simulink model "Integrated_Model"  (R2023b)
settings: Solver=ode23s  StartTime=0.0  StopTime=120  FixedStep=0.01  RelTol=1e-3
undefined symbols (not defined in the file): A_sm, A_stack, A_VGS_center, cmp, cp_coolant, ctrl, estNcr, eta_hex, eta_M, J_rotor, k_e_M, k_t_M, lambda, M_H2O, M_Nmix, M_O2, m_st_Nmix_init, m_st_O2_init, m_st_vp_init, p_amb, p_init, R_init, R_M, R_Nmix, R_O2, R_vp, RH_amb, T_amb, T_coolant, T_init, tbn, V_sm, V_stack, V_tbn_m, yO2_amb
libraries: slpidlib x5
(part 1 of 3)
settings Model: Creator=KOTA-Z  LastModifiedBy=KOTA-Z
settings DataIOCC: SaveFinalState=on  SaveOutput=off  DSMLogging=off

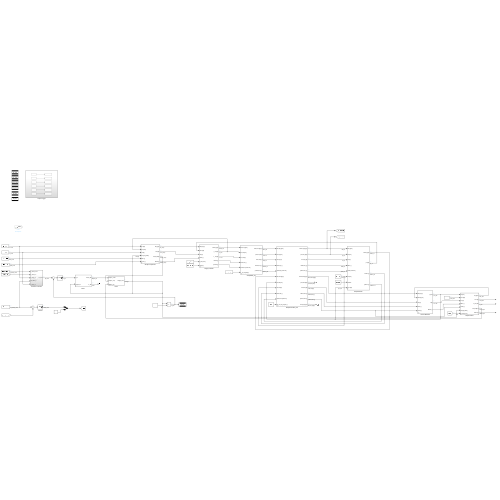
[thumbnail: Simulink's stored preview of the top-level diagram]
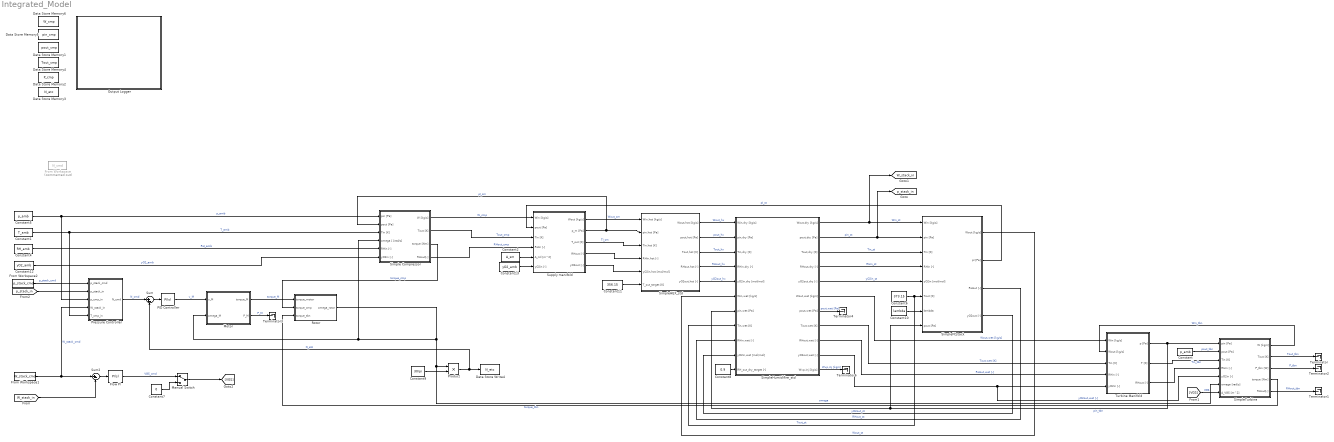
== system Integrated_Model ==
  Constant : Constant  Value=p_amb
  Constant1 : Constant  Value=T_amb
  Constant10 : Constant  Value=lambda
  Constant11 : Constant  Value=356.15
  Constant12 : Constant  Value=yO2_amb
  Constant13 : Constant  Value=yO2_amb
  Constant2 : Constant  Value=A_sm
  Constant4 : Constant  Value=RH_amb
  Constant5 : Constant  Value=p_amb
  Constant6 : Constant  Value=373.15
  Constant7 : Constant  Value=0
  Constant8 : Constant  Value=0.9
  Constant9 : Constant  Value=30/pi
  Data Store Memory1 : DataStoreMemory  DataStoreName=pout_cmp  WriteAfterWriteMsg=warning  ShowAdditionalParam=off
  Data Store Memory2 : DataStoreMemory  DataStoreName=P_cmp  WriteAfterWriteMsg=warning  ShowAdditionalParam=off
  Data Store Memory3 : DataStoreMemory  DataStoreName=N_etc  WriteAfterWriteMsg=warning  ShowAdditionalParam=off
  Data Store Memory4 : DataStoreMemory  DataStoreName=Tout_cmp  WriteAfterWriteMsg=warning  ShowAdditionalParam=off
  Data Store Memory5 : DataStoreMemory  DataStoreName=pin_cmp  WriteAfterWriteMsg=warning  ShowAdditionalParam=off
  Data Store Memory6 : DataStoreMemory  DataStoreName=W_cmp  WriteAfterWriteMsg=warning  ShowAdditionalParam=off
  Data Store Write4 : DataStoreWrite  DataStoreName=N_etc  IndexOptions=Index vector (dialog)  Indices=1  OutputSizes=1
  Flow PI : slpidlib/PID Controller  Controller=PI  Form=Parallel  TimeDomain=Continuous-time  UseExternalTs=off  SampleTime=-1  IntegratorMethod=Forward Euler  FilterMethod=Forward Euler  ControllerParametersSource=internal  P=ctrl.flow.P  I=ctrl.flow.I  UseKiTs=off  D=0  N=100  UseFilter=on  TunerSelectOption=Transfer Function Based (PID Tuner App)  InitialConditionSource=internal  InitialConditionForIntegrator=0  InitialConditionForFilter=0  DifferentiatorICPrevScaledInput=0  ExternalReset=none  TrackingMode=off  Kt=1  LimitOutput=on  SatLimitsSource=internal  UpperSaturationLimit=inf  LowerSaturationLimit=-A_VGS_center  LinearizeAsGain=on  AntiWindupMode=none  Kb=1  LimitIntegrator=off  UpperIntegratorSaturationLimit=inf  LowerIntegratorSaturationLimit=-inf  POutMin=[]  POutMax=[]  IOutMin=[]  IOutMax=[]  DOutMin=[]  DOutMax=[]  NOutMin=[]  NOutMax=[]  SumOutMin=[]  SumOutMax=[]  SaturationOutMin=[]  SaturationOutMax=[]  PParamMin=[]  PParamMax=[]  IParamMin=[]  IParamMax=[]  DParamMin=[]  DParamMax=[]  NParamMin=[]  NParamMax=[]  KbParamMin=[]  KbParamMax=[]  KtParamMin=[]  KtParamMax=[]  KbOutMin=[]  KbOutMax=[]  KtOutMin=[]  KtOutMax=[]  IntegratorOutMin=[]  IntegratorOutMax=[]  FilterOutMin=[]  FilterOutMax=[]  SumI1OutMin=[]  SumI1OutMax=[]  SumI2OutMin=[]  SumI2OutMax=[]  SumI3OutMin=[]  SumI3OutMax=[]  SumI4OutMin=[]  SumI4OutMax=[]  SumDOutMin=[]  SumDOutMax=[]  DifferentiatorOutMin=[]  DifferentiatorOutMax=[]  FilterDiffOutCoefMin=[]  FilterDiffOutCoefMax=[]  ReciprocalOutMin=[]  ReciprocalOutMax=[]  SumDenOutMin=[]  SumDenOutMax=[]  SumNumOutMin=[]  SumNumOutMax=[]  DivideOutMin=[]  DivideOutMax=[]  UdiffTsProdOutMin=[]  UdiffTsProdOutMax=[]  NTsProdOutMin=[]  NTsProdOutMax=[]  UintegralTsProdOutMin=[]  UintegralTsProdOutMax=[]  UngainTsProdOutMin=[]  UngainTsProdOutMax=[]  ClampingZeroOutDataTypeStr=Inherit: Inherit via back propagation  ClampingZeroOutMin=[]  ClampingZeroOutMax=[]  FilterDenConstantOutDataTypeStr=Inherit: Inherit via back propagation  FilterDenConstantOutMin=[]  FilterDenConstantOutMax=[]  PCopyOutDataTypeStr=Inherit: Inherit via back propagation  PCopyOutMin=[]  PCopyOutMax=[]  NCopyOutDataTypeStr=Inherit: Inherit via back propagation  NCopyOutMin=[]  NCopyOutMax=[]  IntegratorContinuousStateAttributes=''  IntegratorStateMustResolveToSignalObject=off  IntegratorRTWStateStorageClass=Auto  FilterContinuousStateAttributes=''  FilterStateMustResolveToSignalObject=off  FilterRTWStateStorageClass=Auto  ParallelPVariant=InternalParameters  IdealPVariant=Disabled  IVariant=InternalParameters  DVariant=Disabled  IntegratorVariant=Continuous  SatVariant=Enabled  AWVariant=Passthrough  PCopyVariant=Disabled  TRVariant=Disabled  FdbkBlocksVariant=Forward  IdealPFdbkVariant=Disabled  SatFdbkVariant=Disabled  DerivativeFilterVariant=Disabled  NVariant=Disabled  NCopyVariant=Disabled_SignalSpec  FilterICVariant=Disabled  IntegratorICVariant=InternalICs  ExternalResetVariant=Disabled  TRSumVariant=Passthrough  SumFdbkVariant=Disabled  SumVariant=Sum_PI  TsampFilterVariant=InternalTs  TsampNgainVariant=Passthrough  TsampIntegralVariant=Disabled_SignalSpec  ExternalSaturationOutDataTypeStr=Inherit: Same as second input
  From Workspace : FromWorkspace  Commented=on  VariableName=N_cmd
  From Workspace1 : FromWorkspace  VariableName=W_stack_cmd
  From Workspace2 : FromWorkspace  VariableName=p_stack_cmd
  Manual Switch : ManualSwitch
  Motor : Subsystem  mask{k_t_M=k_t_M, k_e_M=k_e_M, R_M=R_M, eta_M=eta_M}
      mask prompts: k_t_M "トルク定数 [N*m/A]"; k_e_M "逆起電力係数 [V/(rad/s)]"; R_M "巻線抵抗 [Ω]"; eta_M "モータ機械効率"
      mask DialogControl Parameters Prompt: Motor Parameter
  Output Logger : Subsystem
  PID Controller : slpidlib/PID Controller  Controller=PI  Form=Parallel  TimeDomain=Continuous-time  UseExternalTs=off  SampleTime=-1  IntegratorMethod=Forward Euler  FilterMethod=Forward Euler  ControllerParametersSource=internal  P=ctrl.motor.P  I=ctrl.motor.I  UseKiTs=off  D=0  N=100  UseFilter=on  TunerSelectOption=Transfer Function Based (PID Tuner App)  InitialConditionSource=internal  InitialConditionForIntegrator=0  InitialConditionForFilter=0  DifferentiatorICPrevScaledInput=0  ExternalReset=none  TrackingMode=off  Kt=1  LimitOutput=on  SatLimitsSource=internal  UpperSaturationLimit=500  LowerSaturationLimit=0  LinearizeAsGain=on  AntiWindupMode=none  Kb=1  LimitIntegrator=off  UpperIntegratorSaturationLimit=inf  LowerIntegratorSaturationLimit=-inf  POutMin=[]  POutMax=[]  IOutMin=[]  IOutMax=[]  DOutMin=[]  DOutMax=[]  NOutMin=[]  NOutMax=[]  SumOutMin=[]  SumOutMax=[]  SaturationOutMin=[]  SaturationOutMax=[]  PParamMin=[]  PParamMax=[]  IParamMin=[]  IParamMax=[]  DParamMin=[]  DParamMax=[]  NParamMin=[]  NParamMax=[]  KbParamMin=[]  KbParamMax=[]  KtParamMin=[]  KtParamMax=[]  KbOutMin=[]  KbOutMax=[]  KtOutMin=[]  KtOutMax=[]  IntegratorOutMin=[]  IntegratorOutMax=[]  FilterOutMin=[]  FilterOutMax=[]  SumI1OutMin=[]  SumI1OutMax=[]  SumI2OutMin=[]  SumI2OutMax=[]  SumI3OutMin=[]  SumI3OutMax=[]  SumI4OutMin=[]  SumI4OutMax=[]  SumDOutMin=[]  SumDOutMax=[]  DifferentiatorOutMin=[]  DifferentiatorOutMax=[]  FilterDiffOutCoefMin=[]  FilterDiffOutCoefMax=[]  ReciprocalOutMin=[]  ReciprocalOutMax=[]  SumDenOutMin=[]  SumDenOutMax=[]  SumNumOutMin=[]  SumNumOutMax=[]  DivideOutMin=[]  DivideOutMax=[]  UdiffTsProdOutMin=[]  UdiffTsProdOutMax=[]  NTsProdOutMin=[]  NTsProdOutMax=[]  UintegralTsProdOutMin=[]  UintegralTsProdOutMax=[]  UngainTsProdOutMin=[]  UngainTsProdOutMax=[]  ClampingZeroOutDataTypeStr=Inherit: Inherit via back propagation  ClampingZeroOutMin=[]  ClampingZeroOutMax=[]  FilterDenConstantOutDataTypeStr=Inherit: Inherit via back propagation  FilterDenConstantOutMin=[]  FilterDenConstantOutMax=[]  PCopyOutDataTypeStr=Inherit: Inherit via back propagation  PCopyOutMin=[]  PCopyOutMax=[]  NCopyOutDataTypeStr=Inherit: Inherit via back propagation  NCopyOutMin=[]  NCopyOutMax=[]  IntegratorContinuousStateAttributes=''  IntegratorStateMustResolveToSignalObject=off  IntegratorRTWStateStorageClass=Auto  FilterContinuousStateAttributes=''  FilterStateMustResolveToSignalObject=off  FilterRTWStateStorageClass=Auto  ParallelPVariant=InternalParameters  IdealPVariant=Disabled  IVariant=InternalParameters  DVariant=Disabled  IntegratorVariant=Continuous  SatVariant=Enabled  AWVariant=Passthrough  PCopyVariant=Disabled  TRVariant=Disabled  FdbkBlocksVariant=Forward  IdealPFdbkVariant=Disabled  SatFdbkVariant=Disabled  DerivativeFilterVariant=Disabled  NVariant=Disabled  NCopyVariant=Disabled_SignalSpec  FilterICVariant=Disabled  IntegratorICVariant=InternalICs  ExternalResetVariant=Disabled  TRSumVariant=Passthrough  SumFdbkVariant=Disabled  SumVariant=Sum_PI  TsampFilterVariant=InternalTs  TsampNgainVariant=Passthrough  TsampIntegralVariant=Disabled_SignalSpec  ExternalSaturationOutDataTypeStr=Inherit: Same as second input
  Pressure Controller : Subsystem
  Product : Product
  Rotor : Subsystem  mask{J_rotor=J_rotor}
      mask prompts: J_rotor "Inertia [kg*m^2]"
      mask DialogControl Parameters Prompt: Rotor Parameter
  Simple Compressor : Subsystem  mask{dc=cmp.param.dc, coeff_a=cmp.map.coeff.a, coeff_b=cmp.map.coeff.b, coeff_c=cmp.map.coeff.c, eta_is_cmp=cmp.param.eta_is, eta_m_cmp=cmp.param.eta_mech}
      mask prompts: dc "Inpeller outer diameter"; coeff_a "Map coeffiecient a"; coeff_b "Map coeffiecient b"; coeff_c "Map coeffiecient c"; eta_is_cmp "Isentropic efficiency"; eta_m_cmp "Mechanical efficiency"
      mask DialogControl CmpParameters Prompt: Compressor Parameters
  SimpleFCstack : Subsystem  mask(Simple FCstack){V_ca=V_stack, A_ca=A_stack, R_Nmix=R_Nmix, R_O2=R_O2, R_H2O=R_vp, M_Nmix=M_Nmix, M_O2=M_O2, M_H2O=M_H2O}
      mask prompts: V_ca "Stack Volume (Cathode side) [m^3]"; A_ca "Stack Flow area (Cathode side) [m^2]"; R_Nmix "Gas Constant Nmix [J/kg/K]"; R_O2 "Gas Constant O2 [J/kg/K]"; R_H2O "Gas Constant H2O [J/kg/K]"; M_Nmix "Molecular Weight Nmix [kg/mol]"; M_O2 "Molecular Weight O2 [kg/mol]"; M_H2O "Molecular Weight H2O [kg/mol]"
      mask help: This block provides a simplified FCstack model. The reacted O2 and generated H2O in the stack are calculated based on lambda. Delay due to volume is considered and the pressure drop is approximated as the orifice law.
      mask DialogControl ParameterGroupVar Prompt: Geometric parameter
      mask DialogControl Container3 Prompt: Physical property
  SimpleHEX_std : Subsystem  mask(Simple Heatexchanger){eta_hex=eta_hex, T_cool=T_coolant, cp_cool=cp_coolant}
      mask prompts: eta_hex "Efficiency of HEX [-]"; T_cool "Temperature of coolant [K]"; cp_cool "cp of coolant [J/kg/K]"
      mask help: This block provides a simplified heatexchanger model. Based on the specified thermal efficiency, the exchanged heat is determined.
      mask DialogControl Container3 Prompt: Heatexchanger Parameter
  SimpleHumidifire_std : Subsystem  mask(Simple Humidifire){V_hm=0.1, A_hm=0.1, M_N2=M_Nmix, M_O2=M_O2, M_H2O=M_H2O}
      mask prompts: V_hm "Volume [m^3] (not used)"; A_hm "Flow area [m^2] ] (not used)"; M_N2 "Molecular Weight N2 [kg/mol]"; M_O2 "Molecular Weight O2 [kg/mol]"; M_H2O "Molecular Weight H2O [kg/mol]"
      mask help: This block provides a simplified humidifire model. Depending on the inputed target RH at outlet in dry side, the amount of vapor exchanged between dry and wet side will be calculated. Delay due to volume and pressure drop is not considered.
      mask DialogControl ParameterGroupVar Prompt: Geometric parameter
      mask DialogControl Container3 Prompt: Physical property
  SimpleTurbine : Subsystem  mask{eta_is_tbn=tbn.param.eta_is, eta_m_tbn=tbn.param.eta_mech}
      mask prompts: eta_is_tbn "Isentropic efficiency"; eta_m_tbn "Mechanical efficiency"
      mask DialogControl TbnParameters Prompt: Turbine Parameters
  Sum : Sum  Inputs=|+-
  Sum2 : Sum  Inputs=|+-
  Supply manifold : Subsystem  mask(Supply Manifold){V_m=V_sm, Cd=0.64}
      mask prompts: V_m "Manifold volume [m^3]"; Cd "Discharge coefficient"
      mask help: This block is composed a manifold and a nozzle model.
      mask DialogControl ParameterGroupVar Prompt: Parameter
  Terminator{,1..4,6} (6 alike) : Terminator
  Turbine Manifold : Subsystem  mask{V_m=V_tbn_m}
      mask prompts: V_m "Volume [m^3]"
      mask DialogControl Parameters Prompt: Manifold Parameter
  tag scope: W_stack_in=global, p_stack_in=global
  wires:
  Constant1/1 -> Pressure Controller/5(T_cmp_in), Simple Compressor/3(Tin [K])  "T_amb"
  Constant5/1 -> Pressure Controller/3(p_cmp_in), Simple Compressor/1(pin [Pa])  "p_amb"
  Simple Compressor/1(W [kg/s]) -> Supply manifold/1(Win [kg/s])  "W_cmp"
  Simple Compressor/2(Tout [K]) -> Supply manifold/3(Tin [K])  "Tout_cmp"
  Constant9/1 -> Product/2
  Product/1 -> Sum/2, Data Store Write4/1  "N_etc"
  Rotor/1(omega_rotor) -> Simple Compressor/4(omega [ [rad/s]), Motor/2(omega_M), SimpleTurbine/6(omega [rad/s]), Product/1  "omega"
  Motor/2(P_M) -> Terminator3/1  "P_M"
  Motor/1(torque_M) -> Rotor/1(torque_motor)  "torque_M"
  Simple Compressor/3(torque [Nm]) -> Rotor/2(torque_cmp)  "torque_cmp"
  PID Controller/1 -> Motor/1(v_M)  "v_M"
  Sum/1 -> PID Controller/1
  Constant4/1 -> Simple Compressor/5(RHin [-])  "RH_amb"
  Supply manifold/2(p_m [Pa]) -> SimpleHEX_std/2(pin,hot [Pa]), Simple Compressor/2(pout [Pa])  "pI_sm"
  Constant2/1 -> Supply manifold/5(A_nzl [m^2])
  Simple Compressor/4(RHout[-]) -> Supply manifold/4(RHin [-])  "RHout_cmp"
  SimpleTurbine/1(W [kg/s]) -> Turbine Manifold/2(Wout [kg/s])  "Win_tbn"
  Turbine Manifold/2(T [K]) -> SimpleTurbine/3(Tin [K])  "Tin_tbn"
  Turbine Manifold/1(p [Pa]) -> SimpleFCstack/8(pout [Pa]), SimpleHumidifire_std/7(pin,wet [Pa]), SimpleTurbine/1(pin [Pa])  "pin_tbn"
  Constant/1 -> SimpleTurbine/2(pout [Pa])  "pout_tbn"
  Turbine Manifold/3(RHout [-]) -> SimpleTurbine/4(RHin [-])
  SimpleTurbine/2(Tout [K]) -> Terminator/1  "Tout_tbn"
  SimpleTurbine/5(RHout[-]) -> Terminator1/1  "RHout_tbn"
  SimpleTurbine/3(P_tbn [W]) -> Terminator2/1  "P_tbn"
  Constant10/1 -> SimpleFCstack/7(lambda)
  Supply manifold/1(Wout [kg/s]) -> SimpleHEX_std/1(Win,hot [kg/s])  "Wout_sm"
  Supply manifold/3(T_out [K]) -> SimpleHEX_std/3(Tin,hot [K])  "TI_sm"
  Supply manifold/4(RHout [-]) -> SimpleHEX_std/4(RHin,hot [-])
  SimpleHEX_std/5(yO2out,hot [-]) -> SimpleHumidifire_std/5(yO2in,dry [mol/mol])  "yO2out_hx"
  SimpleHumidifire_std/1(Wout,dry [kg/s]) -> [W_stack_in], SimpleFCstack/1(Win [kg/s])  "Win_st"
  SimpleHumidifire_std/2(pout,dry [Pa]) -> [p_stack_in], SimpleFCstack/2(pin [Pa])  "pin_st"
  SimpleHumidifire_std/3(Tout,dry [K]) -> SimpleFCstack/3(Tin [K])  "Tin_st"
  SimpleHumidifire_std/4(RHout,dry [-]) -> SimpleFCstack/4(RHin [-])  "RHin_st"
  SimpleHumidifire_std/5(yO2out,dry [-]) -> SimpleFCstack/5(yO2in [mol/mol])  "yO2in_st"
  SimpleFCstack/1(Wout [kg/s]) -> SimpleHumidifire_std/6(Win,wet [kg/s])  "Wout_st"
  SimpleFCstack/2(pI [Pa]) -> Supply manifold/2(pout [Pa])  "pI_st"
  Constant6/1 -> SimpleHumidifire_std/8(Tin,wet [K]), SimpleFCstack/6(Tout [K])  "Tout_st"
  SimpleFCstack/3(RHout [-]) -> SimpleHumidifire_std/9(RHin,wet [-])  "RHout_st"
  SimpleFCstack/4(yO2out [-]) -> SimpleHumidifire_std/10(yO2in,wet [mol/mol])  "yO2out_st"
  Constant8/1 -> SimpleHumidifire_std/11(RH_out_dry_target [-])
  SimpleHumidifire_std/6(Wout,wet [kg/s]) -> Turbine Manifold/1(Win [kg/s])  "Wout,wet [kg/s]"
  SimpleHumidifire_std/8(Tout,wet [K]) -> Turbine Manifold/3(Tin [K])  "Tout,wet [K]"
  SimpleHumidifire_std/9(RHout,wet [-]) -> Turbine Manifold/4(RHin [-])  "RHout,wet [-]"
  SimpleTurbine/4(torque [Nm]) -> Rotor/3(torque_tbn)  "torque_tbn"
  SimpleHumidifire_std/7(pout,wet [Pa]) -> Terminator4/1  "pout,wet [Pa]"
  SimpleHumidifire_std/10(yO2out,wet [-]) -> SimpleTurbine/5(yO2in [-]), Turbine Manifold/5(yO2in [-])  "yO2out,wet [-]"
  SimpleHumidifire_std/11(Wvp,inj [kg/s]) -> Terminator6/1  "Wvp,inj [kg/s]"
  Supply manifold/5(yO2out [-]) -> SimpleHEX_std/5(yO2in,hot [mol/mol])
  SimpleHEX_std/3(Tout,hot [K]) -> SimpleHumidifire_std/3(Tin,dry [K])  "Tout_hx"
  SimpleHEX_std/4(RHout,hot [-]) -> SimpleHumidifire_std/4(RHin,dry [-])  "RHout_hx"
  Constant11/1 -> SimpleHEX_std/6(T_out_target [K])
  [VGS] -> SimpleTurbine/7(A_VGS [m^2])  "VGS"
  Sum2/1 -> Flow PI/1
  [W_stack_in] -> Sum2/2
  From Workspace1/1 -> Pressure Controller/4(W_stack_in), Sum2/1  "W_stack_cmd"
  Constant7/1 -> Manual Switch/2
  Manual Switch/1 -> [VGS]
  Flow PI/1 -> Manual Switch/1  "VGS_cmd"
  SimpleHEX_std/1(Wout,hot [kg/s]) -> SimpleHumidifire_std/1(Win,dry [kg/s])  "Wout_hx"
  SimpleHEX_std/2(pout,hot [Pa]) -> SimpleHumidifire_std/2(pin,dry [Pa])  "pout_hx"
  Constant12/1 -> Simple Compressor/6(yO2in [-])  "yO2_amb"
  Constant13/1 -> Supply manifold/6(yO2in [-])
  From Workspace2/1 -> Pressure Controller/1(p_stack_cmd)  "p_stack_cmd"
  [p_stack_in] -> Pressure Controller/2(p_stack_in)
  Pressure Controller/1(N_cmd) -> Sum/1  "N_cmd"

== system Integrated_Model/Motor ==
  v_M : Inport
  omega_M : Inport  Port=2
  Constant : Constant  Value=eta_M*k_t_M/R_M
  Constant1 : Constant  Value=k_e_M
  Minus : Sum  Inputs=+-
  Product : Product
  Product1 : Product
  Product2 : Product
  torque_M : Outport
  P_M : Outport  Port=2
  wires:
  v_M/1 -> Minus/1
  Constant/1 -> Product/2
  Constant1/1 -> Product1/2
  Product1/1 -> Minus/2
  Minus/1 -> Product/1
  omega_M/1 -> Product2/2, Product1/1
  Product/1 -> torque_M/1, Product2/1
  Product2/1 -> P_M/1

== system Integrated_Model/Output Logger ==
  Data Store Read : DataStoreRead  DataStoreName=pin_cmp  IndexOptions=Index vector (dialog)  Indices=1  OutputSizes=1
  Data Store Read1 : DataStoreRead  DataStoreName=W_cmp  IndexOptions=Index vector (dialog)  Indices=1  OutputSizes=1
  Data Store Read2 : DataStoreRead  DataStoreName=Tout_cmp  IndexOptions=Index vector (dialog)  Indices=1  OutputSizes=1
  Data Store Read3 : DataStoreRead  DataStoreName=N_etc  IndexOptions=Index vector (dialog)  Indices=1  OutputSizes=1
  Data Store Read4 : DataStoreRead  DataStoreName=pout_cmp  IndexOptions=Index vector (dialog)  Indices=1  OutputSizes=1
  Data Store Read5 : DataStoreRead  DataStoreName=P_cmp  IndexOptions=Index vector (dialog)  Indices=1  OutputSizes=1
  To Workspace : ToWorkspace  VariableName=pin_cmp  SaveFormat=Timeseries  SampleTime=-1
  To Workspace1 : ToWorkspace  VariableName=pout_cmp  SaveFormat=Timeseries  SampleTime=-1
  To Workspace2 : ToWorkspace  VariableName=W_cmp  SaveFormat=Timeseries  SampleTime=-1
  To Workspace3 : ToWorkspace  VariableName=N_etc  SaveFormat=Timeseries  SampleTime=-1
  To Workspace4 : ToWorkspace  VariableName=Tout_cmp  SaveFormat=Timeseries  SampleTime=-1
  To Workspace5 : ToWorkspace  VariableName=P_cmp  SaveFormat=Timeseries  SampleTime=-1
  wires:
  Data Store Read/1 -> To Workspace/1  "pin_cmp"
  Data Store Read2/1 -> To Workspace4/1
  Data Store Read1/1 -> To Workspace2/1
  Data Store Read4/1 -> To Workspace1/1
  Data Store Read3/1 -> To Workspace3/1
  Data Store Read5/1 -> To Workspace5/1

== system Integrated_Model/Pressure Controller ==
  p_stack_cmd : Inport
  p_stack_in : Inport  Port=2
  p_cmp_in : Inport  Port=3
  W_stack_in : Inport  Port=4
  T_cmp_in : Inport  Port=5
  Display : Display
  Display1 : Display
  Display2 : Display
  Divide : Product  Inputs=*/
  MATLAB Function : MATLAB Function  TreatAsAtomicUnit=on  mask{Ncr_table=estNcr.Ncr_table, Wcr_table=estNcr.Wcr_table, PR_table=estNcr.PR_table}
      mask prompts: Ncr_table "Ncr table [rpm]"; Wcr_table "Wcr table [kg/s]"; PR_table "PR table"
  MATLAB Function1 : MATLAB Function  TreatAsAtomicUnit=on  mask{pref=cmp.ref.p, Tref=cmp.ref.T}
      mask prompts: pref "Refference pressure [Pa]"; Tref "Refference temperature [Pa]"
  MATLAB Function2 : MATLAB Function  TreatAsAtomicUnit=on  mask{Tref=cmp.ref.T}
      mask prompts: Tref "Refference temperature [Pa]"
  Pressure PI : slpidlib/PID Controller  Controller=PI  Form=Parallel  TimeDomain=Continuous-time  UseExternalTs=off  SampleTime=-1  IntegratorMethod=Forward Euler  FilterMethod=Forward Euler  ControllerParametersSource=internal  P=ctrl.pressure.P  I=ctrl.pressure.I  UseKiTs=off  D=0  N=100  UseFilter=on  TunerSelectOption=Transfer Function Based (PID Tuner App)  InitialConditionSource=internal  InitialConditionForIntegrator=0  InitialConditionForFilter=0  DifferentiatorICPrevScaledInput=0  ExternalReset=none  TrackingMode=off  Kt=1  LimitOutput=on  SatLimitsSource=internal  UpperSaturationLimit=20e3  LowerSaturationLimit=-20e3  LinearizeAsGain=on  AntiWindupMode=back-calculation  Kb=1  LimitIntegrator=off  UpperIntegratorSaturationLimit=inf  LowerIntegratorSaturationLimit=-inf  POutMin=[]  POutMax=[]  IOutMin=[]  IOutMax=[]  DOutMin=[]  DOutMax=[]  NOutMin=[]  NOutMax=[]  SumOutMin=[]  SumOutMax=[]  SaturationOutMin=[]  SaturationOutMax=[]  PParamMin=[]  PParamMax=[]  IParamMin=[]  IParamMax=[]  DParamMin=[]  DParamMax=[]  NParamMin=[]  NParamMax=[]  KbParamMin=[]  KbParamMax=[]  KtParamMin=[]  KtParamMax=[]  KbOutMin=[]  KbOutMax=[]  KtOutMin=[]  KtOutMax=[]  IntegratorOutMin=[]  IntegratorOutMax=[]  FilterOutMin=[]  FilterOutMax=[]  SumI1OutMin=[]  SumI1OutMax=[]  SumI2OutMin=[]  SumI2OutMax=[]  SumI3OutMin=[]  SumI3OutMax=[]  SumI4OutMin=[]  SumI4OutMax=[]  SumDOutMin=[]  SumDOutMax=[]  DifferentiatorOutMin=[]  DifferentiatorOutMax=[]  FilterDiffOutCoefMin=[]  FilterDiffOutCoefMax=[]  ReciprocalOutMin=[]  ReciprocalOutMax=[]  SumDenOutMin=[]  SumDenOutMax=[]  SumNumOutMin=[]  SumNumOutMax=[]  DivideOutMin=[]  DivideOutMax=[]  UdiffTsProdOutMin=[]  UdiffTsProdOutMax=[]  NTsProdOutMin=[]  NTsProdOutMax=[]  UintegralTsProdOutMin=[]  UintegralTsProdOutMax=[]  UngainTsProdOutMin=[]  UngainTsProdOutMax=[]  ClampingZeroOutDataTypeStr=Inherit: Inherit via back propagation  ClampingZeroOutMin=[]  ClampingZeroOutMax=[]  FilterDenConstantOutDataTypeStr=Inherit: Inherit via back propagation  FilterDenConstantOutMin=[]  FilterDenConstantOutMax=[]  PCopyOutDataTypeStr=Inherit: Inherit via back propagation  PCopyOutMin=[]  PCopyOutMax=[]  NCopyOutDataTypeStr=Inherit: Inherit via back propagation  NCopyOutMin=[]  NCopyOutMax=[]  IntegratorContinuousStateAttributes=''  IntegratorStateMustResolveToSignalObject=off  IntegratorRTWStateStorageClass=Auto  FilterContinuousStateAttributes=''  FilterStateMustResolveToSignalObject=off  FilterRTWStateStorageClass=Auto  ParallelPVariant=InternalParameters  IdealPVariant=Disabled  IVariant=InternalParameters  DVariant=Disabled  IntegratorVariant=Continuous  SatVariant=Enabled  AWVariant=BackCalculation  PCopyVariant=Disabled  TRVariant=Disabled  FdbkBlocksVariant=Forward  IdealPFdbkVariant=Disabled  SatFdbkVariant=Disabled  DerivativeFilterVariant=Disabled  NVariant=Disabled  NCopyVariant=Disabled_SignalSpec  FilterICVariant=Disabled  IntegratorICVariant=InternalICs  ExternalResetVariant=Disabled  TRSumVariant=Passthrough  SumFdbkVariant=Disabled  SumVariant=Sum_PI  TsampFilterVariant=InternalTs  TsampNgainVariant=Passthrough  TsampIntegralVariant=Disabled_SignalSpec  ExternalSaturationOutDataTypeStr=Inherit: Same as second input
  Sum : Sum  Inputs=|++
  Sum1 : Sum  Inputs=|+-
  N_cmd : Outport
  wires:
  p_stack_in/1 -> Sum1/2
  Sum1/1 -> Pressure PI/1
  Sum/1 -> N_cmd/1
  p_stack_cmd/1 -> Divide/1, Sum1/1
  MATLAB Function1/1(Wcr) -> MATLAB Function/1(Wcr_target), Display2/1
  Divide/1 -> Display1/1, MATLAB Function/2(PR_target)
  MATLAB Function/1(Ncr_est) -> MATLAB Function2/1(Ncr), Display/1
  p_cmp_in/1 -> Divide/2, MATLAB Function1/3(pin)
  W_stack_in/1 -> MATLAB Function1/1(Wact)
  T_cmp_in/1 -> MATLAB Function2/2(Tin), MATLAB Function1/2(Tin)
  Pressure PI/1 -> Sum/1  "N_cmd_FB"
  MATLAB Function2/1(Nact) -> Sum/2  "N_cmd_FF"

== system Integrated_Model/Rotor ==
  torque_motor : Inport
  torque_cmp : Inport  Port=2
  torque_tbn : Inport  Port=3
  Constant : Constant  Value=J_rotor
  Divide : Product  Inputs=*/
  Integrator : Integrator
  Minus : Sum  Inputs=+-+
  omega_rotor : Outport
  wires:
  Constant/1 -> Divide/2
  Divide/1 -> Integrator/1  "dω/dt"
  Integrator/1 -> omega_rotor/1
  torque_motor/1 -> Minus/1
  Minus/1 -> Divide/1
  torque_cmp/1 -> Minus/2
  torque_tbn/1 -> Minus/3

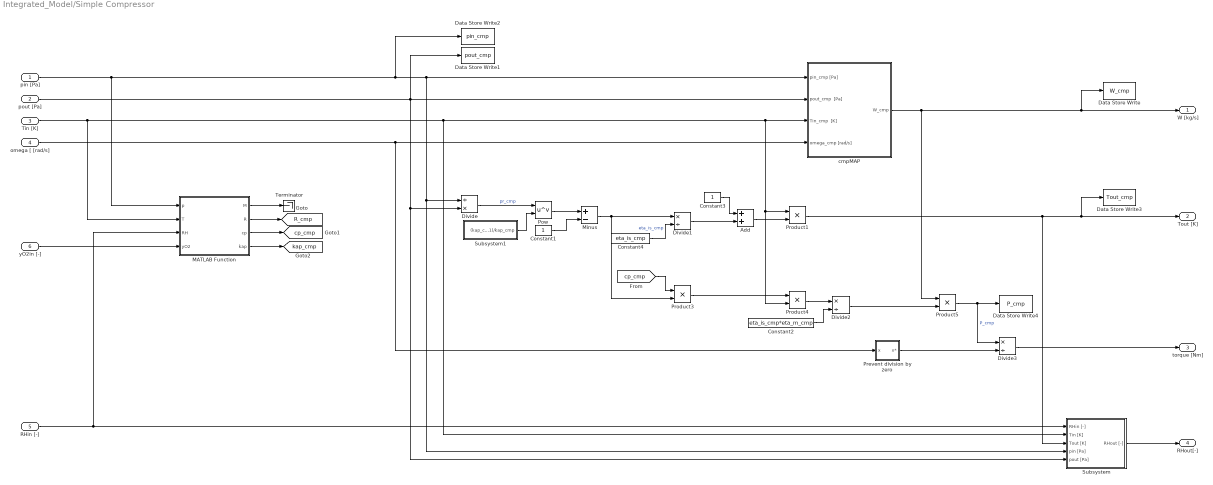
== system Integrated_Model/Simple Compressor ==
  pin [Pa] : Inport
  pout [Pa] : Inport  Port=2
  Tin [K] : Inport  Port=3
  omega [ [rad/s] : Inport  Port=4
  RHin [-] : Inport  Port=5
  yO2in [-] : Inport  Port=6
  Add : Sum
  Constant1 : Constant
  Constant2 : Constant  Value=eta_is_cmp*eta_m_cmp
  Constant3 : Constant
  Constant4 : Constant  Value=eta_is_cmp
  Data Store Write : DataStoreWrite  DataStoreName=W_cmp  IndexOptions=Index vector (dialog)  Indices=1  OutputSizes=1
  Data Store Write1 : DataStoreWrite  DataStoreName=pout_cmp  IndexOptions=Index vector (dialog)  Indices=1  OutputSizes=1
  Data Store Write2 : DataStoreWrite  DataStoreName=pin_cmp  IndexOptions=Index vector (dialog)  Indices=1  OutputSizes=1
  Data Store Write3 : DataStoreWrite  DataStoreName=Tout_cmp  IndexOptions=Index vector (dialog)  Indices=1  OutputSizes=1
  Data Store Write4 : DataStoreWrite  DataStoreName=P_cmp  IndexOptions=Index vector (dialog)  Indices=1  OutputSizes=1
  Divide : Product  Inputs=/*
  Divide1 : Product  Inputs=*/
  Divide2 : Product  Inputs=*/
  Divide3 : Product  Inputs=*/
  MATLAB Function : MATLAB Function  TreatAsAtomicUnit=on  mask{M_O2=M_O2, M_Nmix=M_Nmix, M_H2O=M_H2O}
      mask prompts: M_O2 "Molar mass O2 [kg/mol]"; M_Nmix "Molar mass Nmix [kg/mol]"; M_H2O "Molar mass H2O [kg/mol]"
  Minus : Sum  Inputs=+-
  Pow : Math  Operator=pow  RndMeth=Zero
  Prevent division by zero : Subsystem
  Product{1,3..5} (4 alike) : Product
  Subsystem : Subsystem
  Subsystem1 : Subsystem
  Terminator : Terminator
  cmpMAP : Subsystem
  W [kg/s] : Outport
  Tout [K] : Outport  Port=2
  torque [Nm] : Outport  Port=3
  RHout[-] : Outport  Port=4
  tag scope: R_cmp=global, cp_cmp=global, kap_cmp=global
  wires:
  Divide/1 -> Pow/1  "pr_cmp"
  Subsystem1/1((kap_cmp-1)/kap_cmp) -> Pow/2
  Pow/1 -> Minus/1
  Minus/1 -> Divide1/1, Product3/2
  Constant4/1 -> Divide1/2  "eta_is_cmp"
  Divide1/1 -> Add/2
  Constant3/1 -> Add/1
  Add/1 -> Product1/2
  Tin [K]/1 -> MATLAB Function/2(T), cmpMAP/3(Tin_cmp  [K]), Product4/2, Product1/1, Subsystem/2(Tin [K])
  Constant1/1 -> Minus/2
  [cp_cmp] -> Product3/1
  Product3/1 -> Product4/1
  Product4/1 -> Divide2/1
  Constant2/1 -> Divide2/2
  Divide2/1 -> Product5/2
  Product5/1 -> Data Store Write4/1, Divide3/1  "P_cmp"
  omega [ [rad/s]/1 -> cmpMAP/4(omega_cmp [rad/s]), Prevent division by zero/1(x)
  Prevent division by zero/1(x*) -> Divide3/2
  Divide3/1 -> torque [Nm]/1
  Subsystem/1(RHout [-]) -> RHout[-]/1
  pout [Pa]/1 -> Data Store Write1/1, cmpMAP/2(pout_cmp  [Pa]), Divide/2, Subsystem/5(pout [Pa])
  pin [Pa]/1 -> MATLAB Function/1(p), cmpMAP/1(pin_cmp [Pa]), Divide/1, Subsystem/4(pin [Pa]), Data Store Write2/1
  MATLAB Function/2(R) -> [R_cmp]
  MATLAB Function/3(cp) -> [cp_cmp]
  MATLAB Function/4(kap) -> [kap_cmp]
  MATLAB Function/1(M) -> Terminator/1
  yO2in [-]/1 -> MATLAB Function/4(yO2)
  RHin [-]/1 -> MATLAB Function/3(RH), Subsystem/1(RHin [-])
  cmpMAP/1(W_cmp) -> Product5/1, Data Store Write/1, W [kg/s]/1
  Product1/1 -> Subsystem/3(Tout [K]), Data Store Write3/1, Tout [K]/1

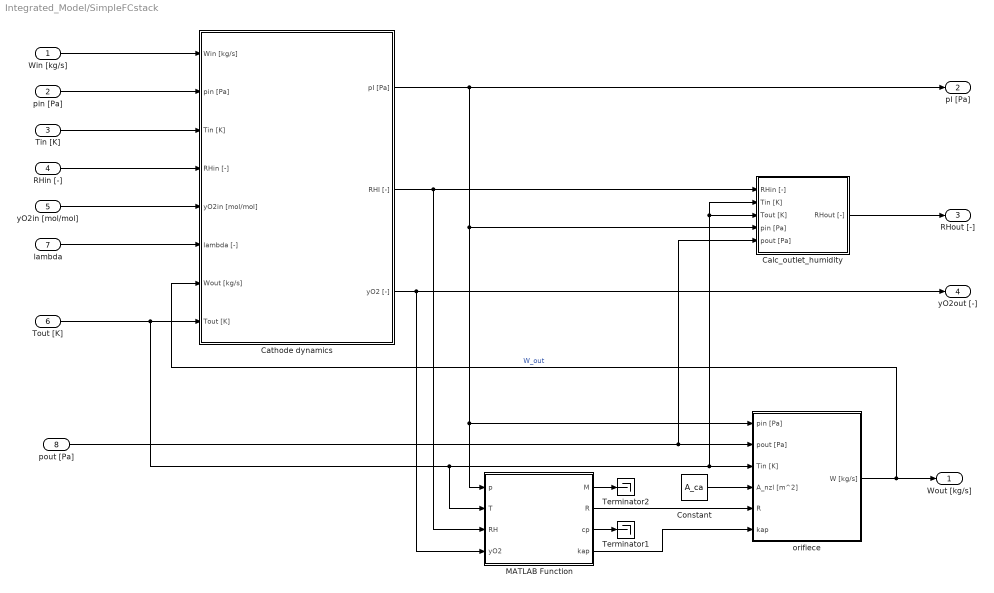
== system Integrated_Model/SimpleFCstack ==
  Win [kg/s] : Inport
  pin [Pa] : Inport  Port=2
  Tin [K] : Inport  Port=3
  RHin [-] : Inport  Port=4
  yO2in [mol/mol] : Inport  Port=5
  Tout [K] : Inport  Port=6
  lambda : Inport  Port=7
  pout [Pa] : Inport  Port=8
  Calc_outlet_humidity : Subsystem
  Cathode dynamics : Subsystem
  Constant : Constant  Value=A_ca
  MATLAB Function : MATLAB Function  TreatAsAtomicUnit=on  mask{M_O2=M_O2, M_Nmix=M_Nmix, M_H2O=M_H2O}
      mask prompts: M_O2 "Molar mass O2 [kg/mol]"; M_Nmix "Molar mass Nmix [kg/mol]"; M_H2O "Molar mass H2O [kg/mol]"
  Terminator1 : Terminator
  Terminator2 : Terminator
  orifiece : Subsystem  mask{Cd_nzl=0.64}
      mask prompts: Cd_nzl "Discharge coefficient"
      mask DialogControl Parameters Prompt: Manifold Parameter
  Wout [kg/s] : Outport
  pI [Pa] : Outport  Port=2
  RHout [-] : Outport  Port=3
  yO2out [-] : Outport  Port=4
  wires:
  pout [Pa]/1 -> orifiece/2(pout [Pa]), Calc_outlet_humidity/5(pout [Pa])
  orifiece/1(W [kg/s]) -> Cathode dynamics/7(Wout [kg/s]), Wout [kg/s]/1  "W_out"
  Constant/1 -> orifiece/4(A_nzl [m^2])
  Cathode dynamics/3(yO2 [-]) -> MATLAB Function/4(yO2), yO2out [-]/1
  Win [kg/s]/1 -> Cathode dynamics/1(Win [kg/s])
  pin [Pa]/1 -> Cathode dynamics/2(pin [Pa])
  lambda/1 -> Cathode dynamics/6(lambda [-])
  Tin [K]/1 -> Cathode dynamics/3(Tin [K])
  RHin [-]/1 -> Cathode dynamics/4(RHin [-])
  Cathode dynamics/1(pI [Pa]) -> pI [Pa]/1, Calc_outlet_humidity/4(pin [Pa]), MATLAB Function/1(p), orifiece/1(pin [Pa])
  yO2in [mol/mol]/1 -> Cathode dynamics/5(yO2in [mol/mol])
  Tout [K]/1 -> MATLAB Function/2(T), Calc_outlet_humidity/3(Tout [K]), Calc_outlet_humidity/2(Tin [K]), orifiece/3(Tin [K]), Cathode dynamics/8(Tout [K])
  Calc_outlet_humidity/1(RHout [-]) -> RHout [-]/1
  MATLAB Function/4(kap) -> orifiece/6(kap)
  MATLAB Function/1(M) -> Terminator2/1
  MATLAB Function/3(cp) -> Terminator1/1
  MATLAB Function/2(R) -> orifiece/5(R)
  Cathode dynamics/2(RHI [-]) -> MATLAB Function/3(RH), Calc_outlet_humidity/1(RHin [-])

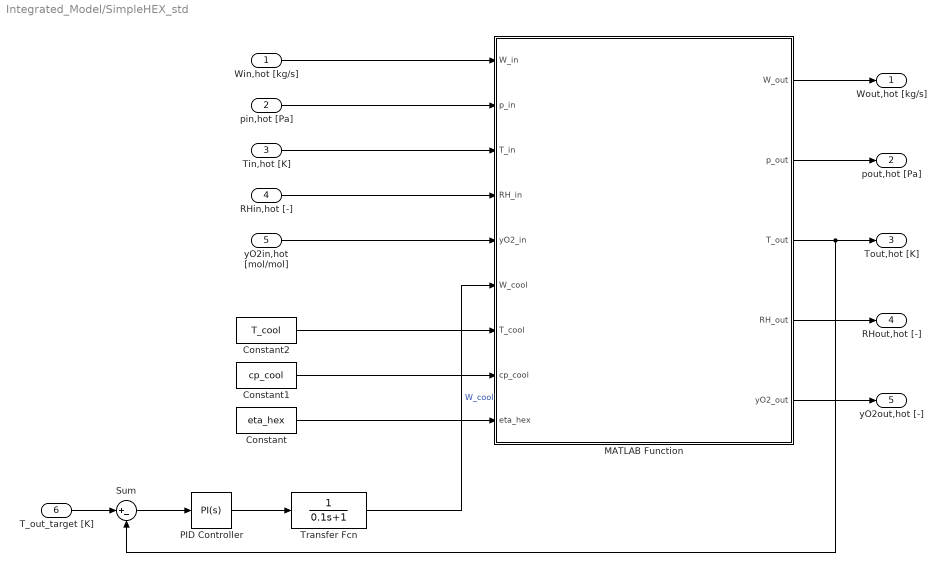
== system Integrated_Model/SimpleHEX_std ==
  Win,hot [kg/s] : Inport
  pin,hot [Pa] : Inport  Port=2
  Tin,hot [K] : Inport  Port=3
  RHin,hot [-] : Inport  Port=4
  yO2in,hot [mol/mol] : Inport  Port=5
  T_out_target [K] : Inport  Port=6
  Constant : Constant  Value=eta_hex
  Constant1 : Constant  Value=cp_cool
  Constant2 : Constant  Value=T_cool
  MATLAB Function : MATLAB Function  TreatAsAtomicUnit=on  mask{M_O2=M_O2, M_Nmix=M_Nmix, M_H2O=M_H2O}
      mask prompts: M_O2 "Molar mass O2 [kg/mol]"; M_Nmix "Molar mass Nmix [kg/mol]"; M_H2O "Molar mass H2O [kg/mol]"
  PID Controller : slpidlib/PID Controller  Controller=PI  Form=Parallel  TimeDomain=Continuous-time  UseExternalTs=off  SampleTime=-1  IntegratorMethod=Forward Euler  FilterMethod=Forward Euler  ControllerParametersSource=internal  P=-0.01  I=-0.1  UseKiTs=off  D=0  N=100  UseFilter=on  TunerSelectOption=Transfer Function Based (PID Tuner App)  InitialConditionSource=internal  InitialConditionForIntegrator=0  InitialConditionForFilter=0  DifferentiatorICPrevScaledInput=0  ExternalReset=none  TrackingMode=off  Kt=1  LimitOutput=on  SatLimitsSource=internal  UpperSaturationLimit=2  LowerSaturationLimit=0  LinearizeAsGain=on  AntiWindupMode=back-calculation  Kb=1  LimitIntegrator=off  UpperIntegratorSaturationLimit=inf  LowerIntegratorSaturationLimit=-inf  POutMin=[]  POutMax=[]  IOutMin=[]  IOutMax=[]  DOutMin=[]  DOutMax=[]  NOutMin=[]  NOutMax=[]  SumOutMin=[]  SumOutMax=[]  SaturationOutMin=[]  SaturationOutMax=[]  PParamMin=[]  PParamMax=[]  IParamMin=[]  IParamMax=[]  DParamMin=[]  DParamMax=[]  NParamMin=[]  NParamMax=[]  KbParamMin=[]  KbParamMax=[]  KtParamMin=[]  KtParamMax=[]  KbOutMin=[]  KbOutMax=[]  KtOutMin=[]  KtOutMax=[]  IntegratorOutMin=[]  IntegratorOutMax=[]  FilterOutMin=[]  FilterOutMax=[]  SumI1OutMin=[]  SumI1OutMax=[]  SumI2OutMin=[]  SumI2OutMax=[]  SumI3OutMin=[]  SumI3OutMax=[]  SumI4OutMin=[]  SumI4OutMax=[]  SumDOutMin=[]  SumDOutMax=[]  DifferentiatorOutMin=[]  DifferentiatorOutMax=[]  FilterDiffOutCoefMin=[]  FilterDiffOutCoefMax=[]  ReciprocalOutMin=[]  ReciprocalOutMax=[]  SumDenOutMin=[]  SumDenOutMax=[]  SumNumOutMin=[]  SumNumOutMax=[]  DivideOutMin=[]  DivideOutMax=[]  UdiffTsProdOutMin=[]  UdiffTsProdOutMax=[]  NTsProdOutMin=[]  NTsProdOutMax=[]  UintegralTsProdOutMin=[]  UintegralTsProdOutMax=[]  UngainTsProdOutMin=[]  UngainTsProdOutMax=[]  ClampingZeroOutDataTypeStr=Inherit: Inherit via back propagation  ClampingZeroOutMin=[]  ClampingZeroOutMax=[]  FilterDenConstantOutDataTypeStr=Inherit: Inherit via back propagation  FilterDenConstantOutMin=[]  FilterDenConstantOutMax=[]  PCopyOutDataTypeStr=Inherit: Inherit via back propagation  PCopyOutMin=[]  PCopyOutMax=[]  NCopyOutDataTypeStr=Inherit: Inherit via back propagation  NCopyOutMin=[]  NCopyOutMax=[]  IntegratorContinuousStateAttributes=''  IntegratorStateMustResolveToSignalObject=off  IntegratorRTWStateStorageClass=Auto  FilterContinuousStateAttributes=''  FilterStateMustResolveToSignalObject=off  FilterRTWStateStorageClass=Auto  ParallelPVariant=InternalParameters  IdealPVariant=Disabled  IVariant=InternalParameters  DVariant=Disabled  IntegratorVariant=Continuous  SatVariant=Enabled  AWVariant=BackCalculation  PCopyVariant=Disabled  TRVariant=Disabled  FdbkBlocksVariant=Forward  IdealPFdbkVariant=Disabled  SatFdbkVariant=Disabled  DerivativeFilterVariant=Disabled  NVariant=Disabled  NCopyVariant=Disabled_SignalSpec  FilterICVariant=Disabled  IntegratorICVariant=InternalICs  ExternalResetVariant=Disabled  TRSumVariant=Passthrough  SumFdbkVariant=Disabled  SumVariant=Sum_PI  TsampFilterVariant=InternalTs  TsampNgainVariant=Passthrough  TsampIntegralVariant=Disabled_SignalSpec  ExternalSaturationOutDataTypeStr=Inherit: Same as second input
  Sum : Sum  Inputs=|+-
  Transfer Fcn : TransferFcn  Denominator=[0.1 1]
  Wout,hot [kg/s] : Outport
  pout,hot [Pa] : Outport  Port=2
  Tout,hot [K] : Outport  Port=3
  RHout,hot [-] : Outport  Port=4
  yO2out,hot [-] : Outport  Port=5
  wires:
  MATLAB Function/5(yO2_out) -> yO2out,hot [-]/1
  MATLAB Function/2(p_out) -> pout,hot [Pa]/1
  MATLAB Function/1(W_out) -> Wout,hot [kg/s]/1
  MATLAB Function/4(RH_out) -> RHout,hot [-]/1
  MATLAB Function/3(T_out) -> Sum/2, Tout,hot [K]/1
  RHin,hot [-]/1 -> MATLAB Function/4(RH_in)
  pin,hot [Pa]/1 -> MATLAB Function/2(p_in)
  Tin,hot [K]/1 -> MATLAB Function/3(T_in)
  Win,hot [kg/s]/1 -> MATLAB Function/1(W_in)
  yO2in,hot [mol/mol]/1 -> MATLAB Function/5(yO2_in)
  PID Controller/1 -> Transfer Fcn/1
  Transfer Fcn/1 -> MATLAB Function/6(W_cool)  "W_cool"
  Sum/1 -> PID Controller/1
  T_out_target [K]/1 -> Sum/1
  Constant2/1 -> MATLAB Function/7(T_cool)
  Constant1/1 -> MATLAB Function/8(cp_cool)
  Constant/1 -> MATLAB Function/9(eta_hex)

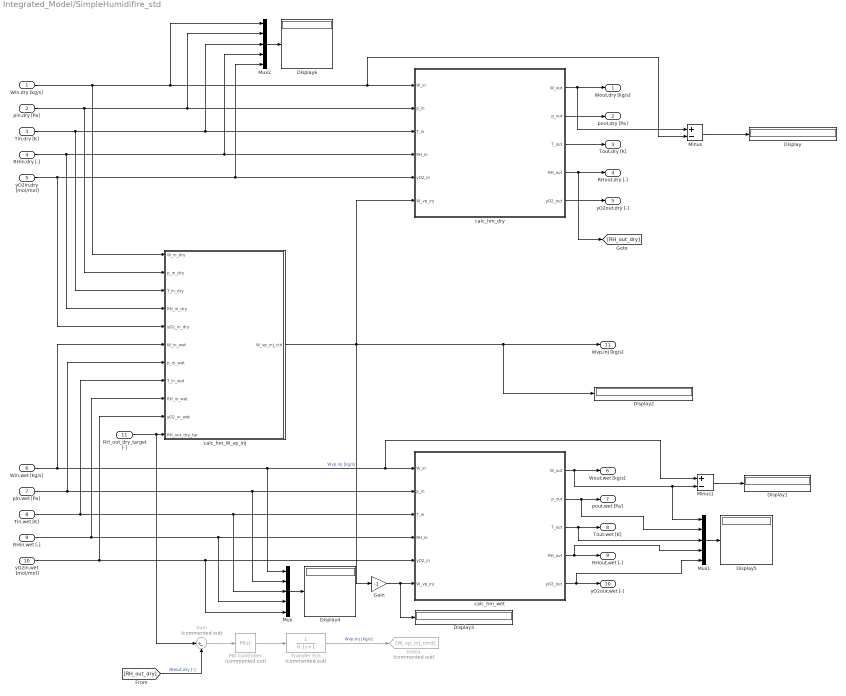
== system Integrated_Model/SimpleHumidifire_std ==
  Win,dry [kg/s] : Inport
  pin,dry [Pa] : Inport  Port=2
  Tin,dry [K] : Inport  Port=3
  RHin,dry [-] : Inport  Port=4
  yO2in,dry [mol/mol] : Inport  Port=5
  Win,wet [kg/s] : Inport  Port=6
  pin,wet [Pa] : Inport  Port=7
  Tin,wet [K] : Inport  Port=8
  RHin,wet [-] : Inport  Port=9
  yO2in,wet [mol/mol] : Inport  Port=10
  RH_out_dry_target [-] : Inport  Port=11
  Display{,1..6} (7 alike) : Display
  Gain : Gain  Gain=-1
  Goto1 : Goto  Commented=on  GotoTag=W_vp_inj_cmd
  Minus : Sum  Inputs=+-
  Minus1 : Sum  Inputs=+-
  Mux : Mux  Inputs=5
  Mux1 : Mux  Inputs=5
  Mux2 : Mux  Inputs=5
  PID Controller : slpidlib/PID Controller  Commented=on  Controller=PI  Form=Parallel  TimeDomain=Continuous-time  UseExternalTs=off  SampleTime=-1  IntegratorMethod=Forward Euler  FilterMethod=Forward Euler  ControllerParametersSource=internal  P=1  I=0.1  UseKiTs=off  D=0  N=100  UseFilter=on  TunerSelectOption=Transfer Function Based (PID Tuner App)  InitialConditionSource=internal  InitialConditionForIntegrator=0  InitialConditionForFilter=0  DifferentiatorICPrevScaledInput=0  ExternalReset=none  TrackingMode=off  Kt=1  LimitOutput=on  SatLimitsSource=internal  UpperSaturationLimit=1  LowerSaturationLimit=0  LinearizeAsGain=on  AntiWindupMode=back-calculation  Kb=1  LimitIntegrator=off  UpperIntegratorSaturationLimit=inf  LowerIntegratorSaturationLimit=-inf  POutMin=[]  POutMax=[]  IOutMin=[]  IOutMax=[]  DOutMin=[]  DOutMax=[]  NOutMin=[]  NOutMax=[]  SumOutMin=[]  SumOutMax=[]  SaturationOutMin=[]  SaturationOutMax=[]  PParamMin=[]  PParamMax=[]  IParamMin=[]  IParamMax=[]  DParamMin=[]  DParamMax=[]  NParamMin=[]  NParamMax=[]  KbParamMin=[]  KbParamMax=[]  KtParamMin=[]  KtParamMax=[]  KbOutMin=[]  KbOutMax=[]  KtOutMin=[]  KtOutMax=[]  IntegratorOutMin=[]  IntegratorOutMax=[]  FilterOutMin=[]  FilterOutMax=[]  SumI1OutMin=[]  SumI1OutMax=[]  SumI2OutMin=[]  SumI2OutMax=[]  SumI3OutMin=[]  SumI3OutMax=[]  SumI4OutMin=[]  SumI4OutMax=[]  SumDOutMin=[]  SumDOutMax=[]  DifferentiatorOutMin=[]  DifferentiatorOutMax=[]  FilterDiffOutCoefMin=[]  FilterDiffOutCoefMax=[]  ReciprocalOutMin=[]  ReciprocalOutMax=[]  SumDenOutMin=[]  SumDenOutMax=[]  SumNumOutMin=[]  SumNumOutMax=[]  DivideOutMin=[]  DivideOutMax=[]  UdiffTsProdOutMin=[]  UdiffTsProdOutMax=[]  NTsProdOutMin=[]  NTsProdOutMax=[]  UintegralTsProdOutMin=[]  UintegralTsProdOutMax=[]  UngainTsProdOutMin=[]  UngainTsProdOutMax=[]  ClampingZeroOutDataTypeStr=Inherit: Inherit via back propagation  ClampingZeroOutMin=[]  ClampingZeroOutMax=[]  FilterDenConstantOutDataTypeStr=Inherit: Inherit via back propagation  FilterDenConstantOutMin=[]  FilterDenConstantOutMax=[]  PCopyOutDataTypeStr=Inherit: Inherit via back propagation  PCopyOutMin=[]  PCopyOutMax=[]  NCopyOutDataTypeStr=Inherit: Inherit via back propagation  NCopyOutMin=[]  NCopyOutMax=[]  IntegratorContinuousStateAttributes=''  IntegratorStateMustResolveToSignalObject=off  IntegratorRTWStateStorageClass=Auto  FilterContinuousStateAttributes=''  FilterStateMustResolveToSignalObject=off  FilterRTWStateStorageClass=Auto  ParallelPVariant=InternalParameters  IdealPVariant=Disabled  IVariant=InternalParameters  DVariant=Disabled  IntegratorVariant=Continuous  SatVariant=Enabled  AWVariant=BackCalculation  PCopyVariant=Disabled  TRVariant=Disabled  FdbkBlocksVariant=Forward  IdealPFdbkVariant=Disabled  SatFdbkVariant=Disabled  DerivativeFilterVariant=Disabled  NVariant=Disabled  NCopyVariant=Disabled_SignalSpec  FilterICVariant=Disabled  IntegratorICVariant=InternalICs  ExternalResetVariant=Disabled  TRSumVariant=Passthrough  SumFdbkVariant=Disabled  SumVariant=Sum_PI  TsampFilterVariant=InternalTs  TsampNgainVariant=Passthrough  TsampIntegralVariant=Disabled_SignalSpec  ExternalSaturationOutDataTypeStr=Inherit: Same as second input
  Sum : Sum  Commented=on  Inputs=|+-
  Transfer Fcn : TransferFcn  Commented=on  Denominator=[0.1 1]
  calc_hm_W_vp_inj : MATLAB Function  TreatAsAtomicUnit=on  mask{M_O2=M_O2, M_Nmix=M_Nmix, M_H2O=M_H2O}
      mask prompts: M_O2 "Molar mass O2 [kg/mol]"; M_Nmix "Molar mass N2 [kg/mol]"; M_H2O "Molar mass H2O [kg/mol]"
  calc_hm_dry : MATLAB Function  TreatAsAtomicUnit=on  mask{M_O2=M_O2, M_Nmix=M_Nmix, M_H2O=M_H2O}
      mask prompts: M_O2 "Molar mass O2 [kg/mol]"; M_Nmix "Molar mass Nmix [kg/mol]"; M_H2O "Molar mass H2O [kg/mol]"
  calc_hm_wet : MATLAB Function  TreatAsAtomicUnit=on  mask{M_O2=M_O2, M_Nmix=M_Nmix, M_H2O=M_H2O}
      mask prompts: M_O2 "Molar mass O2 [kg/mol]"; M_Nmix "Molar mass Nmix [kg/mol]"; M_H2O "Molar mass H2O [kg/mol]"
  Wout,dry [kg/s] : Outport
  pout,dry [Pa] : Outport  Port=2
  Tout,dry [K] : Outport  Port=3
  RHout,dry [-] : Outport  Port=4
  yO2out,dry [-] : Outport  Port=5
  Wout,wet [kg/s] : Outport  Port=6
  pout,wet [Pa] : Outport  Port=7
  Tout,wet [K] : Outport  Port=8
  RHout,wet [-] : Outport  Port=9
  yO2out,wet [-] : Outport  Port=10
  Wvp,inj [kg/s] : Outport  Port=11
  wires:
  calc_hm_dry/5(yO2_out) -> yO2out,dry [-]/1
  calc_hm_dry/2(p_out) -> pout,dry [Pa]/1
  calc_hm_dry/4(RH_out) -> RHout,dry [-]/1, [RH_out_dry]
  calc_hm_dry/3(T_out) -> Tout,dry [K]/1
  pin,wet [Pa]/1 -> Mux/2, calc_hm_wet/2(p_in), calc_hm_W_vp_inj/7(p_in_wet)
  Win,wet [kg/s]/1 -> Mux/1, calc_hm_wet/1(W_in), Minus1/1, calc_hm_W_vp_inj/6(W_in_wet)
  RHin,wet [-]/1 -> Mux/4, calc_hm_wet/4(RH_in), calc_hm_W_vp_inj/9(RH_in_wet)
  yO2in,wet [mol/mol]/1 -> Mux/5, calc_hm_wet/5(yO2_in), calc_hm_W_vp_inj/10(yO2_in_wet)
  Tin,wet [K]/1 -> Mux/3, calc_hm_wet/3(T_in), calc_hm_W_vp_inj/8(T_in_wet)
  calc_hm_wet/1(W_out) -> Mux1/1, Minus1/2, Wout,wet [kg/s]/1
  calc_hm_wet/2(p_out) -> Mux1/2, pout,wet [Pa]/1
  calc_hm_wet/3(T_out) -> Mux1/3, Tout,wet [K]/1
  calc_hm_wet/4(RH_out) -> Mux1/4, RHout,wet [-]/1
  calc_hm_wet/5(yO2_out) -> Mux1/5, yO2out,wet [-]/1
  PID Controller/1 -> Transfer Fcn/1
  Transfer Fcn/1 -> Goto1/1  "Wvp,inj [kg/s]"
  Sum/1 -> PID Controller/1
  RH_out_dry_target [-]/1 -> calc_hm_W_vp_inj/11(RH_out_dry_tar), Sum/1
  [RH_out_dry] -> Sum/2  "RHout,dry [-]"
  Gain/1 -> Display3/1, calc_hm_wet/6(W_vp_inj)
  calc_hm_W_vp_inj/1(W_vp_inj_ctrl) -> calc_hm_dry/6(W_vp_inj), Display2/1, Wvp,inj [kg/s]/1, Gain/1  "Wvp,inj [kg/s]"
  Minus/1 -> Display/1
  calc_hm_dry/1(W_out) -> Minus/1, Wout,dry [kg/s]/1
  Minus1/1 -> Display1/1
  Mux/1 -> Display4/1
  Mux1/1 -> Display5/1
  pin,dry [Pa]/1 -> Mux2/2, calc_hm_dry/2(p_in), calc_hm_W_vp_inj/2(p_in_dry)
  Tin,dry [K]/1 -> Mux2/3, calc_hm_dry/3(T_in), calc_hm_W_vp_inj/3(T_in_dry)
  Win,dry [kg/s]/1 -> Mux2/1, Minus/2, calc_hm_dry/1(W_in), calc_hm_W_vp_inj/1(W_in_dry)
  RHin,dry [-]/1 -> Mux2/4, calc_hm_dry/4(RH_in), calc_hm_W_vp_inj/4(RH_in_dry)
  yO2in,dry [mol/mol]/1 -> Mux2/5, calc_hm_dry/5(yO2_in), calc_hm_W_vp_inj/5(yO2_in_dry)
  Mux2/1 -> Display6/1

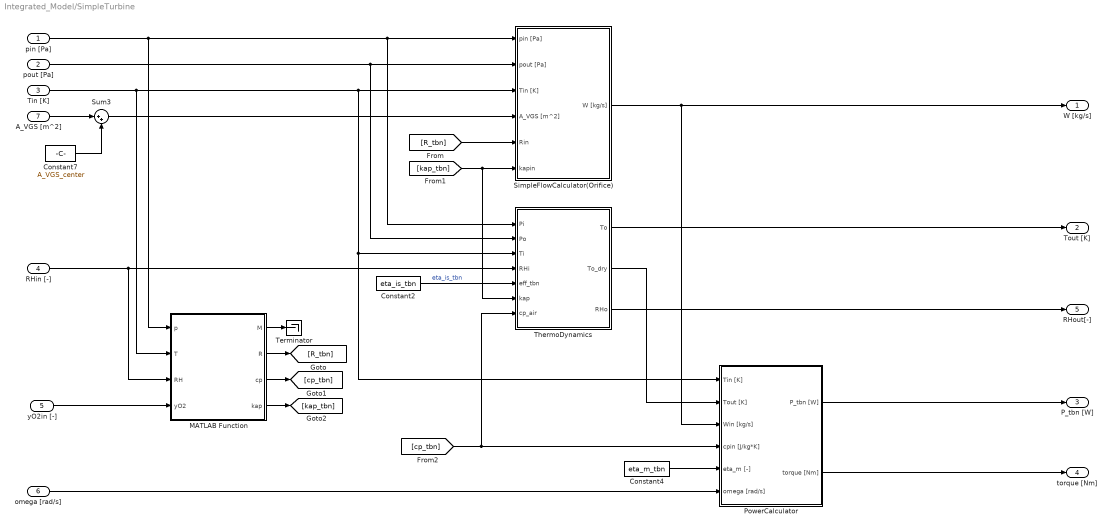
== system Integrated_Model/SimpleTurbine ==
  pin [Pa] : Inport
  pout [Pa] : Inport  Port=2
  Tin [K] : Inport  Port=3
  RHin [-] : Inport  Port=4
  yO2in [-] : Inport  Port=5
  omega [rad/s] : Inport  Port=6
  A_VGS [m^2] : Inport  Port=7
  Constant2 : Constant  Value=eta_is_tbn
  Constant4 : Constant  Value=eta_m_tbn
  Constant7 : Constant  Value=A_VGS_center
  MATLAB Function : MATLAB Function  TreatAsAtomicUnit=on  mask{M_O2=M_O2, M_Nmix=M_Nmix, M_H2O=M_H2O}
      mask prompts: M_O2 "Molar mass O2 [kg/mol]"; M_Nmix "Molar mass Nmix [kg/mol]"; M_H2O "Molar mass H2O [kg/mol]"
  PowerCalculator : Subsystem
  SimpleFlowCalculator(Orifice) : Subsystem
  Sum3 : Sum  Inputs=|++
  Terminator : Terminator
  ThermoDynamics : MATLAB Function  TreatAsAtomicUnit=on
  W [kg/s] : Outport
  Tout [K] : Outport  Port=2
  P_tbn [W] : Outport  Port=3
  torque [Nm] : Outport  Port=4
  RHout[-] : Outport  Port=5
  wires:
  pin [Pa]/1 -> MATLAB Function/1(p), ThermoDynamics/1(Pi), SimpleFlowCalculator(Orifice)/1(pin [Pa])
  Tin [K]/1 -> MATLAB Function/2(T), SimpleFlowCalculator(Orifice)/3(Tin [K]), PowerCalculator/1(Tin [K]), ThermoDynamics/3(Ti)
  SimpleFlowCalculator(Orifice)/1(W [kg/s]) -> PowerCalculator/3(Win [kg/s]), W [kg/s]/1
  pout [Pa]/1 -> ThermoDynamics/2(Po), SimpleFlowCalculator(Orifice)/2(pout [Pa])
  ThermoDynamics/3(RHo) -> RHout[-]/1
  PowerCalculator/1(P_tbn [W]) -> P_tbn [W]/1
  [R_tbn] -> SimpleFlowCalculator(Orifice)/5(Rin)
  [kap_tbn] -> ThermoDynamics/6(kap), SimpleFlowCalculator(Orifice)/6(kapin)
  Constant4/1 -> PowerCalculator/5(eta_m [-])
  omega [rad/s]/1 -> PowerCalculator/6(omega [rad/s])
  PowerCalculator/2(torque [Nm]) -> torque [Nm]/1
  Sum3/1 -> SimpleFlowCalculator(Orifice)/4(A_VGS [m^2])
  ThermoDynamics/1(To) -> Tout [K]/1
  Constant2/1 -> ThermoDynamics/5(eff_tbn)  "eta_is_tbn"
  [cp_tbn] -> ThermoDynamics/7(cp_air), PowerCalculator/4(cpin [J/kg*K])
  ThermoDynamics/2(To_dry) -> PowerCalculator/2(Tout [K])
  A_VGS [m^2]/1 -> Sum3/1
  Constant7/1 -> Sum3/2
  MATLAB Function/2(R) -> [R_tbn]
  MATLAB Function/4(kap) -> [kap_tbn]
  MATLAB Function/3(cp) -> [cp_tbn]
  MATLAB Function/1(M) -> Terminator/1
  RHin [-]/1 -> MATLAB Function/3(RH), ThermoDynamics/4(RHi)
  yO2in [-]/1 -> MATLAB Function/4(yO2)

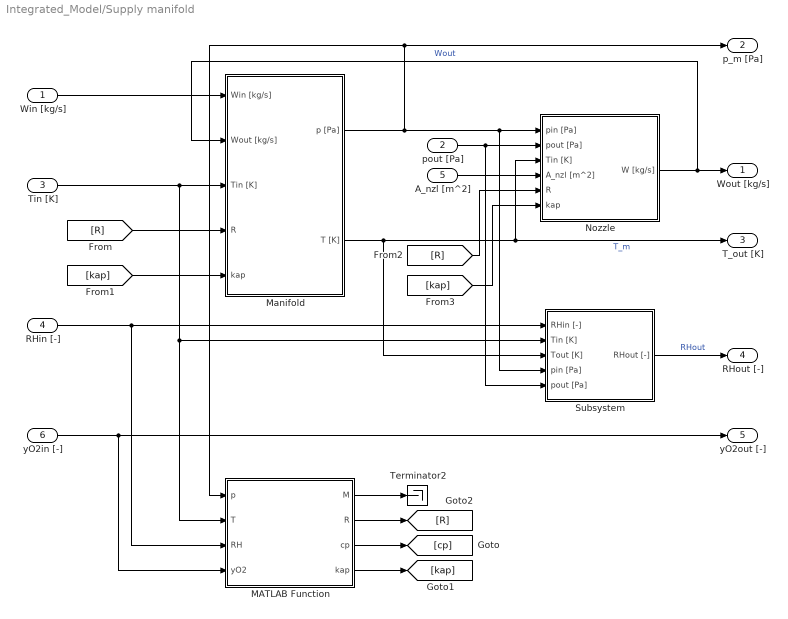
== system Integrated_Model/Supply manifold ==
  Win [kg/s] : Inport
  pout [Pa] : Inport  Port=2
  Tin [K] : Inport  Port=3
  RHin [-] : Inport  Port=4
  A_nzl [m^2] : Inport  Port=5
  yO2in [-] : Inport  Port=6
  MATLAB Function : MATLAB Function  TreatAsAtomicUnit=on  mask{M_O2=M_O2, M_Nmix=M_Nmix, M_H2O=M_H2O}
      mask prompts: M_O2 "Molar mass O2 [kg/mol]"; M_Nmix "Molar mass Nmix [kg/mol]"; M_H2O "Molar mass H2O [kg/mol]"
  Manifold : Subsystem  mask{V_m=V_m}
      mask prompts: V_m "Volume [m^3]"
      mask DialogControl Parameters Prompt: Manifold Parameter
  Nozzle : Subsystem  mask{Cd_nzl=Cd}
      mask prompts: Cd_nzl "Discharge coefficient"
      mask DialogControl Parameters Prompt: Manifold Parameter
  Subsystem : Subsystem
  Terminator2 : Terminator
  Wout [kg/s] : Outport
  p_m [Pa] : Outport  Port=2
  T_out [K] : Outport  Port=3
  RHout [-] : Outport  Port=4
  yO2out [-] : Outport  Port=5
  wires:
  Win [kg/s]/1 -> Manifold/1(Win [kg/s])
  Manifold/2(T [K]) -> Nozzle/3(Tin [K]), T_out [K]/1, Subsystem/3(Tout [K])  "T_m"
  Subsystem/1(RHout [-]) -> RHout [-]/1  "RHout"
  Nozzle/1(W [kg/s]) -> Manifold/2(Wout [kg/s]), Wout [kg/s]/1  "Wout"
  pout [Pa]/1 -> Subsystem/5(pout [Pa]), Nozzle/2(pout [Pa])
  A_nzl [m^2]/1 -> Nozzle/4(A_nzl [m^2])
  yO2in [-]/1 -> MATLAB Function/4(yO2), yO2out [-]/1
  Manifold/1(p [Pa]) -> MATLAB Function/1(p), p_m [Pa]/1, Nozzle/1(pin [Pa]), Subsystem/4(pin [Pa])
  MATLAB Function/4(kap) -> [kap]
  MATLAB Function/2(R) -> [R]
  RHin [-]/1 -> MATLAB Function/3(RH), Subsystem/1(RHin [-])
  MATLAB Function/3(cp) -> [cp]
  MATLAB Function/1(M) -> Terminator2/1
  Tin [K]/1 -> MATLAB Function/2(T), Subsystem/2(Tin [K]), Manifold/3(Tin [K])
  [R] -> Manifold/4(R)
  [kap] -> Manifold/5(kap)
  [R] -> Nozzle/5(R)
  [kap] -> Nozzle/6(kap)

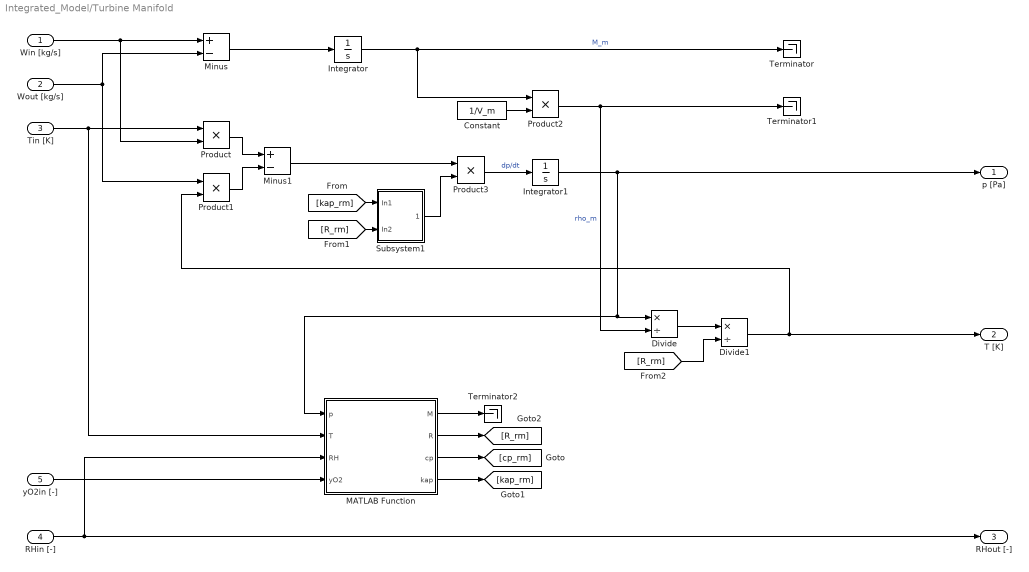
== system Integrated_Model/Turbine Manifold ==
  Win [kg/s] : Inport
  Wout [kg/s] : Inport  Port=2
  Tin [K] : Inport  Port=3
  RHin [-] : Inport  Port=4
  yO2in [-] : Inport  Port=5
  Constant : Constant  Value=1/V_m
  Divide : Product  Inputs=*/
  Divide1 : Product  Inputs=*/
  Integrator : Integrator  InitialCondition=p_init*V_m/(R_init*T_init)
  Integrator1 : Integrator  InitialCondition=p_init
  MATLAB Function : MATLAB Function  TreatAsAtomicUnit=on  mask{M_O2=M_O2, M_Nmix=M_Nmix, M_H2O=M_H2O}
      mask prompts: M_O2 "Molar mass O2 [kg/mol]"; M_Nmix "Molar mass Nmix [kg/mol]"; M_H2O "Molar mass H2O [kg/mol]"
  Minus : Sum  Inputs=+-
  Minus1 : Sum  Inputs=+-
  Product{,1..3} (4 alike) : Product
  Subsystem1 : Subsystem
  Terminator : Terminator
  Terminator1 : Terminator
  Terminator2 : Terminator
  p [Pa] : Outport
  T [K] : Outport  Port=2
  RHout [-] : Outport  Port=3
  wires:
  Win [kg/s]/1 -> Minus/1, Product/2
  Wout [kg/s]/1 -> Product1/1, Minus/2
  Minus/1 -> Integrator/1
  Integrator/1 -> Product2/1, Terminator/1  "M_m"
  Product2/1 -> Terminator1/1, Divide/2  "rho_m"
  Tin [K]/1 -> MATLAB Function/2(T), Product/1
  Product/1 -> Minus1/1
  Product1/1 -> Minus1/2
  Minus1/1 -> Product3/1
  Constant/1 -> Product2/2
  Integrator1/1 -> p [Pa]/1, MATLAB Function/1(p), Divide/1
  [R_rm] -> Divide1/2
  Divide1/1 -> T [K]/1, Product1/2
  Divide/1 -> Divide1/1
  Product3/1 -> Integrator1/1  "dp/dt"
  RHin [-]/1 -> MATLAB Function/3(RH), RHout [-]/1
  yO2in [-]/1 -> MATLAB Function/4(yO2)
  MATLAB Function/1(M) -> Terminator2/1
  MATLAB Function/3(cp) -> [cp_rm]
  MATLAB Function/4(kap) -> [kap_rm]
  MATLAB Function/2(R) -> [R_rm]
  [kap_rm] -> Subsystem1/1(In1)
  [R_rm] -> Subsystem1/2(In2)
  Subsystem1/1(kap*R/V) -> Product3/2

== system Integrated_Model/Simple Compressor/Prevent division by zero ==
  note: ※ゼロ除算防止 : x* = sqrt(x^2 + xth^2)
  x : Inport
  Add : Sum
  Constant4 : Constant  Value=0.01^2
  Sqrt : Sqrt
  Square1 : Math  Operator=square
  x* : Outport
  wires:
  Constant4/1 -> Add/2
  Square1/1 -> Add/1
  x/1 -> Square1/1
  Add/1 -> Sqrt/1
  Sqrt/1 -> x*/1

== system Integrated_Model/Simple Compressor/Subsystem ==
  note: ※凝縮が生じない場合の分圧比はモル分率に等しい
  RHin [-] : Inport
  Tin [K] : Inport  Port=2
  Tout [K] : Inport  Port=3
  pin [Pa] : Inport  Port=4
  pout [Pa] : Inport  Port=5
  Divide : Product  Inputs=*/
  Divide1 : Product  Inputs=*/
  MATLAB Function : MATLAB Function  TreatAsAtomicUnit=on
  MATLAB Function1 : MATLAB Function  TreatAsAtomicUnit=on
  Product : Product
  Product1 : Product
  Terminator : Terminator
  RHout [-] : Outport
  wires:
  MATLAB Function/1(psat) -> Product/2
  Tin [K]/1 -> MATLAB Function/1(Ts)
  Tout [K]/1 -> MATLAB Function1/1(Ts)
  RHin [-]/1 -> Product/1
  Product/1 -> Terminator/1, Divide/1  "pin,vp"
  pin [Pa]/1 -> Divide/2
  Divide/1 -> Product1/1  "pin,vp/pin"
  pout [Pa]/1 -> Product1/2
  Product1/1 -> Divide1/1  "pout,vp"
  MATLAB Function1/1(psat) -> Divide1/2
  Divide1/1 -> RHout [-]/1

== system Integrated_Model/Simple Compressor/Subsystem1 ==
  Constant5 : Constant
  Divide4 : Product  Inputs=*/
  Minus1 : Sum  Inputs=+-
  (kap_cmp-1)/kap_cmp : Outport
  wires:
  [kap_cmp] -> Divide4/2, Minus1/1
  Divide4/1 -> (kap_cmp-1)/kap_cmp/1
  Constant5/1 -> Minus1/2
  Minus1/1 -> Divide4/1

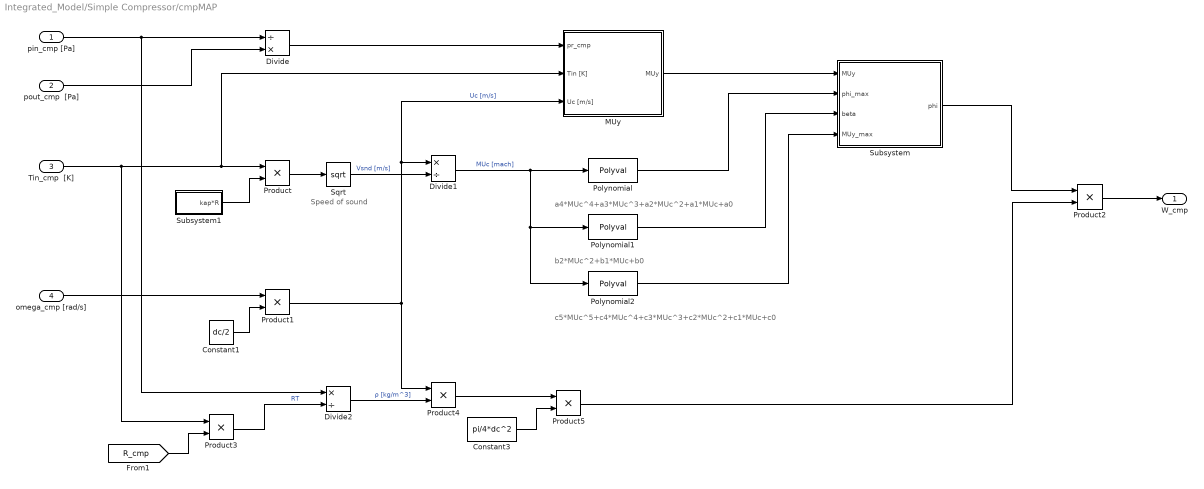
== system Integrated_Model/Simple Compressor/cmpMAP ==
  note: a4*MUc^4+a3*MUc^3+a2*MUc^2+a1*MUc+a0
  note: Speed of sound
  note: b2*MUc^2+b1*MUc+b0
  note: c5*MUc^5+c4*MUc^4+c3*MUc^3+c2*MUc^2+c1*MUc+c0
  pin_cmp [Pa] : Inport
  pout_cmp  [Pa] : Inport  Port=2
  Tin_cmp  [K] : Inport  Port=3
  omega_cmp [rad/s] : Inport  Port=4
  Constant1 : Constant  Value=dc/2
  Constant3 : Constant  Value=pi/4*dc^2
  Divide : Product  Inputs=/*
  Divide1 : Product  Inputs=*/
  Divide2 : Product  Inputs=*/
  MUy : Subsystem
  Polynomial : Polyval  Coefs=coeff_a
  Polynomial1 : Polyval  Coefs=coeff_b
  Polynomial2 : Polyval  Coefs=coeff_c
  Product{,1..5} (6 alike) : Product
  Sqrt : Sqrt
  Subsystem : Subsystem
  Subsystem1 : Subsystem
  W_cmp : Outport
  wires:
  pin_cmp [Pa]/1 -> Divide2/1, Divide/1
  pout_cmp  [Pa]/1 -> Divide/2
  Tin_cmp  [K]/1 -> Product3/1, MUy/2(Tin [K]), Product/1
  Subsystem1/1(kap*R) -> Product/2
  Product/1 -> Sqrt/1
  omega_cmp [rad/s]/1 -> Product1/1
  Constant1/1 -> Product1/2
  Sqrt/1 -> Divide1/2  "Vsnd [m/s]"
  Product1/1 -> MUy/3(Uc [m/s]), Divide1/1, Product4/1  "Uc [m/s]"
  Divide1/1 -> Polynomial/1, Polynomial2/1, Polynomial1/1  "MUc [mach]"
  Divide/1 -> MUy/1(pr_cmp)
  Polynomial/1 -> Subsystem/2(phi_max)
  MUy/1(MUy) -> Subsystem/1(MUy)
  Polynomial1/1 -> Subsystem/3(beta)
  Polynomial2/1 -> Subsystem/4(MUy_max)
  Product2/1 -> W_cmp/1
  Subsystem/1(phi) -> Product2/1
  [R_cmp] -> Product3/2
  Product3/1 -> Divide2/2  "RT"
  Divide2/1 -> Product4/2  "ρ [kg/m^3]"
  Product4/1 -> Product5/1
  Constant3/1 -> Product5/2
  Product5/1 -> Product2/2
